simulink model "mass_spring"  (R2021a)
settings: Solver=VariableStepAuto  StartTime=0.0  StopTime=100  RelTol=1e-3
InitFcn:
  | mass_spring_model
undefined symbols (not defined in the file or in its folder): A, B, C_real, D, K
PostSaveFcn:
  | mass_spring_model
settings Model: PacingRate=9  Creator=umut  LastModifiedBy=umut

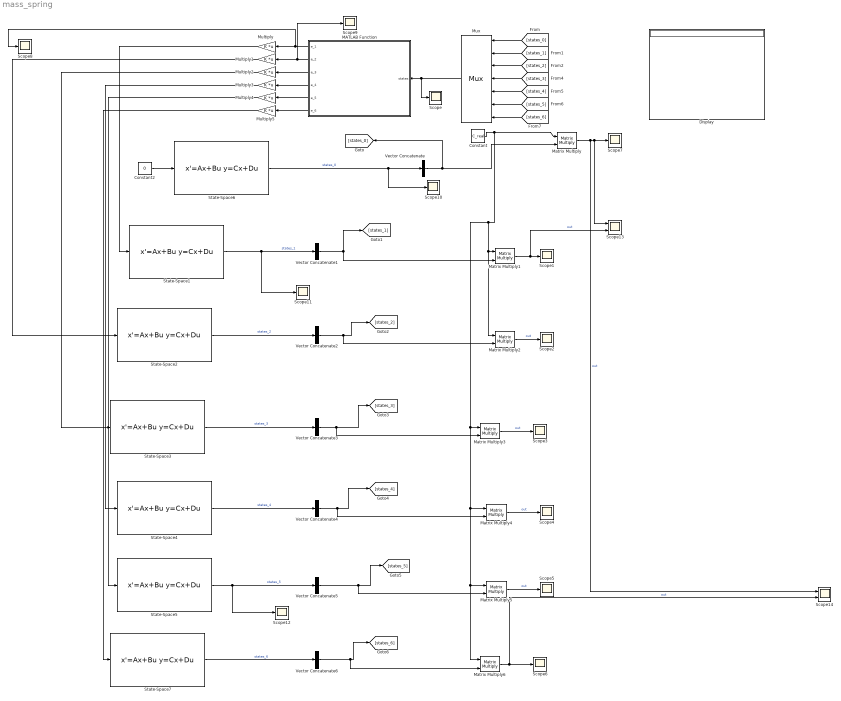
== system mass_spring ==
  Constant : Constant  Value=C_real
  Constant2 : Constant  Value=0
  Display : Display
  MATLAB Function : MATLAB Function  TreatAsAtomicUnit=on
  Matrix Multiply{,1..6} (7 alike) : Product  Multiplication=Matrix(*)
  Multiply{,1..5} (6 alike) : Gain  Gain=K  Multiplication=Matrix(K*u)
  Mux : Mux  Inputs=7
  Scope{,1..12} (13 alike) : Scope
  Scope13 : Scope  NumInputPorts=2
  Scope14 : Scope  NumInputPorts=2
  State-Space{1..4} (4 alike) : StateSpace  A=A  B=B  C=eye(4)  D=D  InitialCondition=0
  State-Space5 : StateSpace  A=A  B=B  C=eye(4)  D=D  InitialCondition=[1;3;4;7]
  State-Space6 : StateSpace  A=A  B=B  C=eye(4)  D=D  InitialCondition=[1;2;3;4]
  State-Space7 : StateSpace  A=A  B=B  C=eye(4)  D=D  InitialCondition=[1,2,3,4]
  Vector Concatenate{,1..6} (7 alike) : Concatenate  NumInputs=1  Mode=Multidimensional array  ConcatenateDimension=4
  wires:
  Matrix Multiply1/1 -> Scope13/2, Scope1/1  "out"
  State-Space1/1 -> Scope11/1, Vector Concatenate1/1  "states_1"
  Mux/1 -> Scope/1, MATLAB Function/1(states)
  State-Space2/1 -> Vector Concatenate2/1  "states_2"
  Matrix Multiply2/1 -> Scope2/1  "out"
  Matrix Multiply3/1 -> Scope3/1  "out"
  State-Space3/1 -> Vector Concatenate3/1  "states_3"
  Matrix Multiply4/1 -> Scope4/1  "out"
  State-Space4/1 -> Vector Concatenate4/1  "states_4"
  Matrix Multiply5/1 -> Scope5/1  "out"
  State-Space5/1 -> Scope12/1, Vector Concatenate5/1  "states_5"
  Matrix Multiply6/1 -> Scope14/2, Scope6/1  "out"
  State-Space7/1 -> Vector Concatenate6/1  "states_6"
  [states_0] -> Mux/1
  [states_1] -> Mux/2
  [states_6] -> Mux/7
  [states_5] -> Mux/6
  [states_4] -> Mux/5
  [states_3] -> Mux/4
  [states_2] -> Mux/3
  MATLAB Function/1(e_1) -> Scope8/1, Multiply/1
  MATLAB Function/2(e_2) -> Scope9/1, Multiply1/1
  MATLAB Function/3(e_3) -> Multiply2/1
  MATLAB Function/4(e_4) -> Multiply3/1
  MATLAB Function/5(e_5) -> Multiply4/1
  MATLAB Function/6(e_6) -> Multiply5/1
  Multiply/1 -> State-Space1/1
  Multiply1/1 -> State-Space2/1
  Multiply2/1 -> State-Space3/1
  Multiply3/1 -> State-Space4/1
  Multiply4/1 -> State-Space5/1
  Multiply5/1 -> State-Space7/1
  Constant/1 -> Matrix Multiply/1, Matrix Multiply6/1, Matrix Multiply5/1, Matrix Multiply4/1, Matrix Multiply3/1, Matrix Multiply2/1, Matrix Multiply1/1
  State-Space6/1 -> Scope10/1, Vector Concatenate/1  "states_0"
  Constant2/1 -> State-Space6/1
  Vector Concatenate/1 -> [states_0], Matrix Multiply/2
  Matrix Multiply/1 -> Scope14/1, Scope13/1, Scope7/1  "out"
  Vector Concatenate1/1 -> Matrix Multiply1/2, [states_1]
  Vector Concatenate2/1 -> Matrix Multiply2/2, [states_2]
  Vector Concatenate3/1 -> Matrix Multiply3/2, [states_3]
  Vector Concatenate4/1 -> Matrix Multiply4/2, [states_4]
  Vector Concatenate5/1 -> Matrix Multiply5/2, [states_5]
  Vector Concatenate6/1 -> Matrix Multiply6/2, [states_6]

== matlab function mass_spring/MATLAB Function ==
  data: states input; e_1 output size=[4, 1]; e_2 output size=[4, 1]; e_3 output size=[4, 1]; e_4 output size=[4, 1]; e_5 output size=[4, 1]; e_6 output size=[4, 1]
function [e_1, e_2, e_3, e_4, e_5, e_6]  = calculate_neighborhood_error(states)
    adj = [ 0	0	0	0	0	0
        2	0	0	0	0	0
        0	6	0	0	0	0
        0	0	1	0	0	0
        0	0	0	1	0	0
        0	0	0	0	3	0];
    
    pinnings = [1; 0; 0; 0; 0; 0];

    A = adj;
    G = pinnings;
    
    size_agents = 6;
    size_states = 4;
    
    error = zeros(size_states, size_agents);
    
    
    for i = 1 : size_agents
        error_temp = [0;0;0;0];
        for j = 1 : size_agents
            error_temp = error_temp + A(i, j) * (states((j)*4+1 : 4*(j+1)) - states((i)*4+1 : 4*(i+1)));
        end
        error_temp = error_temp + pinnings(i) * (states(1 : 4) - states((i)*4+1 : 4*(i+1)));
        error(:,i) = error_temp;
    end
    
    e_1 = error(:,1);
    e_2 = error(:,2);
    e_3 = error(:,3);
    e_4 = error(:,4);
    e_5 = error(:,5);
    e_6 = error(:,6);

end
